simulink model "lorenz"  (R2018b)
settings: Solver=VariableStepAuto  StartTime=0.0  StopTime=60  RelTol=1e-8
settings Model: Creator=1  LastModifiedBy=1
settings DebuggingCC: LibraryContextMissingDiagnostic=none
settings SFSimCC: SimUseLocalCustomCode=off
settings RTWCC: RTWUseLocalCustomCode=off

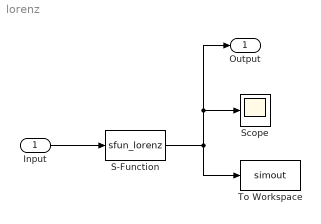
== system lorenz ==
  Input : Inport
  S-Function : S-Function  FunctionName=sfun_lorenz  Parameters=x0, P  SFunctionDeploymentMode=off  EnableBusSupport=off
  Scope : Scope
  To Workspace : ToWorkspace  VariableName=simout  SaveFormat=Timeseries  SampleTime=-1
  Output : Outport
  wires:
  Input/1 -> S-Function/1
  S-Function/1 -> To Workspace/1, Output/1, Scope/1
